simulink model "es1b"  (R2022b)
settings: Solver=VariableStepAuto  StartTime=0.0  StopTime=10.0  RelTol=1e-3
undefined symbols (not defined in the file): A, Ad, B, Bd, C, Cd, D, Dd, den, Kd, Ki, Kp, num, T, Tl
settings Model: Creator=emanuelevitetta  LastModifiedBy=emanuelevitetta

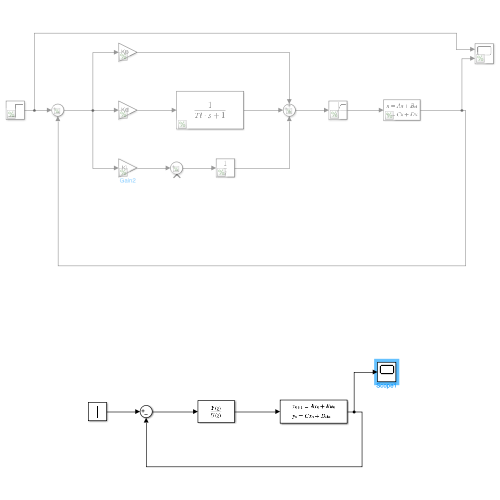
[thumbnail: Simulink's stored preview of the top-level diagram]
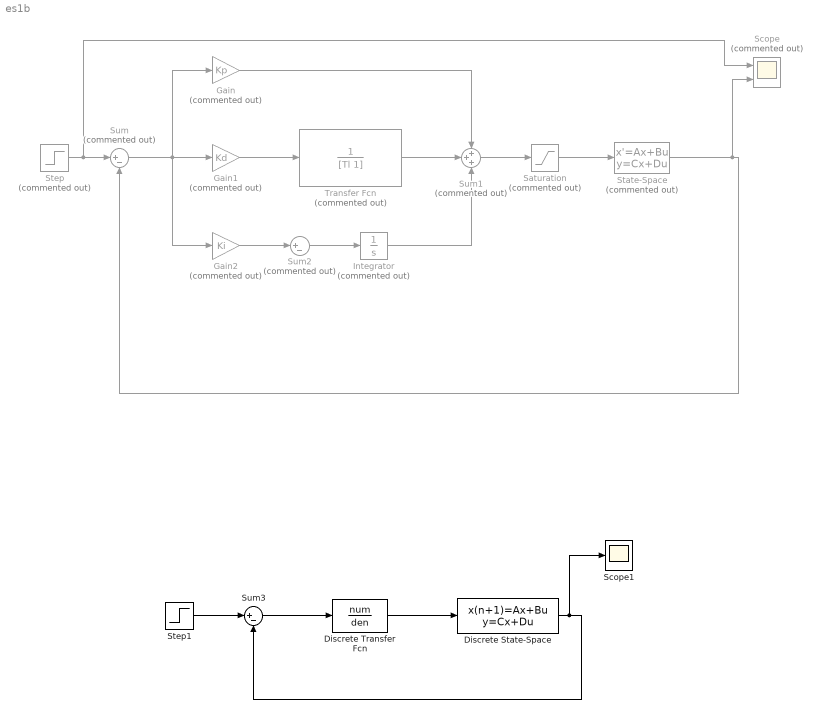
== system es1b ==
  Discrete Transfer Fcn : DiscreteTransferFcn  Numerator=num  Denominator=den  SampleTime=T
  Discrete State-Space : DiscreteStateSpace  A=Ad  B=Bd  C=Cd  D=Dd  SampleTime=T
  Gain : Gain  Commented=on  Gain=Kp
  Gain1 : Gain  Commented=on  Gain=Kd
  Gain2 : Gain  Commented=on  Gain=Ki
  Integrator : Integrator  Commented=on
  Saturation : Saturate  Commented=on  UpperLimit=u  LowerLimit=-u  LinearizeAsGain=off  ZeroCross=off
  Scope : Scope  Commented=on  NumInputPorts=2
  Scope1 : Scope
  State-Space : StateSpace  Commented=on  A=A  B=B  C=C  D=D  InitialCondition=0
  Step : Step  Commented=on  SampleTime=0
  Step1 : Step  SampleTime=0
  Sum : Sum  Commented=on  Inputs=|+-
  Sum1 : Sum  Commented=on  Inputs=+++
  Sum2 : Sum  Commented=on  Inputs=|+-
  Sum3 : Sum  Inputs=|+-
  Transfer Fcn : TransferFcn  Commented=on  Denominator=[Tl 1]
  wires:
  Gain1/1 -> Transfer Fcn/1
  Transfer Fcn/1 -> Sum1/2
  Gain/1 -> Sum1/1
  Gain2/1 -> Sum2/1
  Sum2/1 -> Integrator/1
  Integrator/1 -> Sum1/3
  State-Space/1 -> Scope/2, Sum/2
  Step/1 -> Scope/1, Sum/1
  Sum/1 -> Gain/1, Gain2/1, Gain1/1
  Sum1/1 -> Saturation/1
  Saturation/1 -> State-Space/1
  Step1/1 -> Sum3/1
  Discrete Transfer Fcn/1 -> Discrete State-Space/1
  Sum3/1 -> Discrete Transfer Fcn/1
  Discrete State-Space/1 -> Scope1/1, Sum3/2
